simulink model "MotGenEvDynamic"  (R2021a)
settings: Solver=VariableStepAuto  StartTime=0.0  StopTime=inf  RelTol=1e-3  EnableMultiTasking=on
model workspace (MAT data in the model file):
  EV_current = 200
  EV_motion = [20 4 0.8]
  EV_sf = 2000
  Fs = 0
  Fv = 0.0025
  Jcomp = 0.0227
  Ki = 251.3274
  Kisa = 346.6583
  Kp_d = 0.47149
  Kp_q = 0.52125
  Ksa = 85.4316
  Ksf = 1996.2651
  Ld = 0.000125
  Ldq = [0.000125 0.00013]
  Lq = 0.00013
  Mechanical = [0.0227 0.0025 0]
  P = 4
  PolePairs = 10
  Rs = 0.012
  T_eff_bp = [20 40 60 80 100 120]
  T_max = 100
  T_mtpa = [0 13.3131834767 26.6278836885 39.9456159322 53.2678926341 66.5962219318 79.9321062746 93.277041051 106.632513247 120.000000141]
  ba = 3.4029
  bp = 10
  efficiency_table = [88  90  92  92  92  88; 88  94  95  96  95  94; 88  94  96  96  95  94; 88  94  95  96  95  94; 88  90  94  95  94  94]
  id_mtpa = [0 -0.114523352646 -0.457989076459 -1.03008464374 -1.83029075221 -2.85788367342 -4.11193850568 -5.59133329791 -7.29475400168 -9.22070020138]
  idq0 = [0 0]
  idq_limits = [-9.220699542 166.993501392 167.247872355]
  iq_mtpa = [0 18.5827440345 37.1633719111 55.7397734896 74.3098506185 92.871523015 111.422734008 129.961456105 148.485696337 166.993501356]
  lambda_pm = 0.0393
  mechanical = [0.0227 0.0025 0]
  omega_init = 0
  theta_init = 0
  w_eff_bp = [105 210 315 420 525]
libraries: autolibmotorctrlr x1, autolibpmsminterior x1, autolibinverter x1
settings Model: ModifiedByFormat=The MathWorks, Inc.  SimulationMode=accelerator  PauseTimes=10  Creator=The MathWorks, Inc.  LastModifiedBy=The MathWorks, Inc.
settings SolverCC: AlgebraicLoopSolver=TrustRegion  DecoupledContinuousIntegration=on
settings DataIOCC: DSMLogging=off  ReturnWorkspaceOutputs=off
settings DebuggingCC: UnderspecifiedInitializationDetection=Classic  MergeDetectMultiDrivingBlocksExec=none  SFMachineParentedDataDiag=warning  ArithmeticOperatorsInVariantConditions=warning
settings ModelReferenceCC: PropagateSignalLabelsOutOfModel=off
settings SFSimCC: SimUseLocalCustomCode=off  CustomCodeUndefinedFunction=UseInterfaceOnly
settings RTWCC: RTWUseLocalCustomCode=off
settings CodeAppCC: StateflowObjectComments=on
settings GRTTargetCC: TargetLangStandard=C89/C90 (ANSI)
settings ConfigComp: CovMetricSettings=dsw  CovSaveCumulativeToWorkspaceVar=on  CovSaveSingleToWorkspaceVar=on  CovExternalEMLEnable=off
settings SimscapeCC: SimscapeNormalizeSystem=off

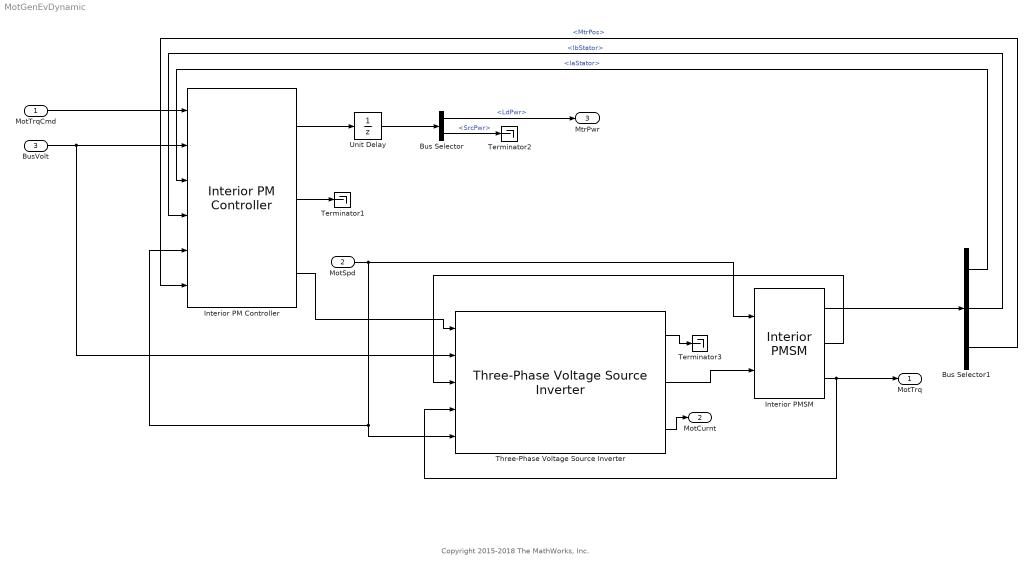
== system MotGenEvDynamic ==
  note: Copyright 2015-2018 The MathWorks, Inc.
  MotTrqCmd : Inport
  MotSpd : Inport  Port=2
  BusVolt : Inport  Port=3
  Bus Selector : BusSelector  OutputSignals=LdPwr,SrcPwr
  Bus Selector1 : BusSelector  OutputSignals=IaStator,IbStator,MtrPos
  Interior PM Controller : autolibmotorctrlr/Interior PM Controller  control_type=Torque Control  Rs=Rs  Ld=Ld  Lq=Lq  lambda_pm=lambda_pm  PolePairs=PolePairs  Mechanical=[0.0027, 4.924e-4, 0]  T_max=T_max  bp=bp  T_mtpa=[0 11.1085586386239 22.2173088185054 33.326442053384 44.4361498019826 55.546623440547 66.6580542354434 77.7706333158326 88.8845516464394 100.000000000437]  id_mtpa=[0 -0.0451770397636582 -0.180701927673943 -0.406555973884657 -0.722708042968231 -1.12911457536488 -1.62571961736212 -2.21245485956083 -2.88923968375932 -3.65598121818655]  iq_mtpa=[0 18.8439267008685 37.6875285035227 56.5304806497674 75.3724586612817 94.2131384791491 113.052196602898 131.889310228892 150.724157387918 169.556417081793]  idq_limits=[-3.65598121132496 169.556417081941 169.595827697154]  EV_current=200  Tst=5e-5  Kp_d=0.15708  Kp_q=0.16336  Ki=15.0796  EV_motion=[20, 4, 0.8]  EV_sf=200  ba=0.40475  Ksa=10.1615  Kisa=41.2325  Ksf=1217.9727  Jcomp=0.0027  Fv=0.0004924  Fs=0  param_loss=Tabulated efficiency data  eff=98  w_loss_bp=[0 200 400 600 800 1000]  T_loss_bp=[0 25 50 75 100]  losses_table=[100 100 100 100 100;100 150 200 250 300;100 200 300 400 500;100 250 400 550 700;100 300 500 700 900;100 350 600 850 1100]  w_eff_bp=w_eff_bp  T_eff_bp=T_eff_bp  efficiency_table=efficiency_table  x_w_bp=[-525 -420 -315 -210 -105 105 210 315 420 525]  x_T_bp=[-120 -100 -80 -60 -40 -20 20 40 60 80 100 120]  x_losses_mat=[4021.27659574468 3351.06382978723 2210.52631578947 2010.63829787234 2333.33333333333 1431.81818181818 1260 2100 1890 2100 3150 3780;3217.02127659574 2210.52631578947 1400 1326.31578947368 1072.34042553191 1145.45454545455 1008 1008 1260 1344 2100 3024;2412.76595744681 1657.8947368421 1050 787.500000000001 804.255319148936 859.09090909091 756 755.999999999999 756.000000000001 1008 1575 2268;1608.51063829787 1105.26315789474 700.000000000001 663.157894736841 536.170212765957 572.727272727273 504 503.999999999999 629.999999999999 672.000000000001 1050 1512;1718.18181818182 913.043478260869 730.434782608695 547.826086956521 466.666666666667 286.363636363637 252 420 504 672 840 1512;1512 840 672 504 420 252 286.363636363637 466.666666666667 547.826086956521 730.434782608695 913.043478260869 1718.18181818182;1512 1050 672.000000000001 629.999999999999 503.999999999999 504 572.727272727273 536.170212765957 663.157894736841 700.000000000001 1105.26315789474 1608.51063829787;2268 1575 1008 756.000000000001 755.999999999999 756 859.09090909091 804.255319148936 787.500000000001 1050 1657.8947368421 2412.76595744681;3024 2100 1344 1260 1008 1008 1145.45454545455 1072.34042553191 1326.31578947368 1400 2210.52631578947 3217.02127659574;3780 3150 2100 1890 2100 1260 1431.81818181818 2333.33333333333 2010.63829787234 2210.52631578947 3351.06382978723 4021.27659574468]  Tsm=5e-4
      settings: SourceProductBaseCode=PW
  Interior PMSM : autolibpmsminterior/Interior PMSM  port_config=Speed  sim_type=Continuous  Ts=0.001  P=PolePairs  Rs=Rs  Ldq=Ldq  KConstText=Permanent flux linkage constant (lambda_pm):  lambda_pm=lambda_pm  Ke=159.9771  mechanical=[0.0027, 4.924e-4, 0]  idq0=[0 0]  theta_init=0  omega_init=0  KConst=lambda_pm  lambda_pm_calc=lambda_pm  Kt=1.323  RefBlkName='autolibpmsminterior/Interior PMSM'  aMode=1
      settings: SourceProductBaseCode=PW,DR,MT,UV,VE
  Terminator1 : Terminator
  Terminator2 : Terminator
  Terminator3 : Terminator
  Three-Phase Voltage Source Inverter : autolibinverter/Three-Phase Voltage Source Inverter  InvrtrTmpInpEnbl=off  enable_hdl=off  model_type=Commanded phase voltage  fs=5000  w_eff_bp=w_eff_bp  n1=128  T_eff_bp=T_eff_bp  Temp_eff_bp=[213.15 293.15 373.15]  n2=128  ploss_table=.97*ones(5,6)  ploss_table_3d=cat(3,0.95*[1 0.999 0.989 0.997 0.996;0.995 0.994 0.993 0.992 0.991;0.990 0.989 0.988 0.987 0.986;0.985 0.984 0.983 0.982 0.981;0.980 0.979 0.978 0.977 0.976],[1 0.999 0.989 0.997 0.996;0.995 0.994 0.993 0.992 0.991;0.990 0.989 0.988 0.987 0.986;0.985 0.984 0.983 0.982 0.981;0.980 0.979 0.978 0.977 0.976],0.92*[1 0.999 0.989 0.997 0.996;0.995 0.994 0.993 0.992 0.991;0.990 0.989 0.988 0.987 0.986;0.985 0.984 0.983 0.982 0.981;0.980 0.979 0.978 0.977 0.976])  preExtrapFlag=off  u1max=1000  u1min=-1000  u2max=200  u2min=-200  intPrec=23  RefBlkName='autolibmappedmotor/Mapped Motor'  CalLossMapData={'BaseCageProjectFileName','';'BaseMbcProjectFileName','MbcPrj_1.mat';'TaskName','Calibrate Inverter Loss Map';'ChildTasks',{{'DataName','';'TaskName','Import Loss Data'},{'TaskName','Generate Response Models'},{'TaskName','Generate Calibration'},{'TaskName','Update Block Parameters'}}}  CalLossWithTempMapData={}
      settings: SourceProductBaseCode=PW,DR,MT,UV,VE
  Unit Delay : UnitDelay  SampleTime=-1  HasFrameUpgradeWarning=on
  MotTrq : Outport  VectorParamsAs1DForOutWhenUnconnected=off
  MotCurnt : Outport  Port=2  VectorParamsAs1DForOutWhenUnconnected=off
  MtrPwr : Outport  Port=3
  wires:
  MotTrqCmd/1 -> Interior PM Controller/1
  BusVolt/1 -> Interior PM Controller/2, Three-Phase Voltage Source Inverter/2
  Bus Selector1/1 -> Interior PM Controller/3  "<IaStator>"
  Interior PMSM/1 -> Bus Selector1/1
  Bus Selector1/3 -> Interior PM Controller/6  "<MtrPos>"
  Bus Selector1/2 -> Interior PM Controller/4  "<IbStator>"
  MotSpd/1 -> Interior PMSM/1, Interior PM Controller/5, Three-Phase Voltage Source Inverter/5
  Interior PM Controller/2 -> Terminator1/1
  Interior PM Controller/1 -> Unit Delay/1
  Three-Phase Voltage Source Inverter/2 -> Interior PMSM/2
  Three-Phase Voltage Source Inverter/1 -> Terminator3/1
  Interior PMSM/2 -> Three-Phase Voltage Source Inverter/3
  Interior PM Controller/3 -> Three-Phase Voltage Source Inverter/1
  Interior PMSM/3 -> Three-Phase Voltage Source Inverter/4, MotTrq/1
  Three-Phase Voltage Source Inverter/3 -> MotCurnt/1
  Bus Selector/1 -> MtrPwr/1  "<LdPwr>"
  Bus Selector/2 -> Terminator2/1  "<SrcPwr>"
  Unit Delay/1 -> Bus Selector/1
